simulink model "pendel_polar"  (Simulink 7.0)
settings: Solver=ode45  StartTime=0.0  StopTime=tstop  FixedStep=0.8  MaxStep=0.8  RelTol=1e-6
values from neighbouring files (symbols this model uses):
  g = 9.81    [main_pendel_kartesisch.m]    (also in main_pendel_polar.m)
  l = 1    [main_pendel_kartesisch.m]    (also in main_pendel_polar.m)
  omega0 = 0    [main_pendel_polar.m]
  phi0 = 45 *pi/180    (= 0.785398163397)    [main_pendel_polar.m]
libraries: simulink x3
settings Model: Creator=adminus  LastModifiedBy=adminus
settings DataIOCC: OutputOption=SpecifiedOutputTimes  OutputTimes=[0:0.01:5]
settings OptimizationCC: BlockReduction=off
settings DebuggingCC: SaveWithParameterizedLinksMsg=none  SignalResolutionControl=TryResolveAllWithWarning  SolverPrmCheckMsg=none  MultiTaskDSMMsg=warning  MultiTaskCondExecSysMsg=none  StrictBusMsg=None
settings HardwareCC: TargetUnknown=on
settings RTWCC: IncludeERTFirstTime=on

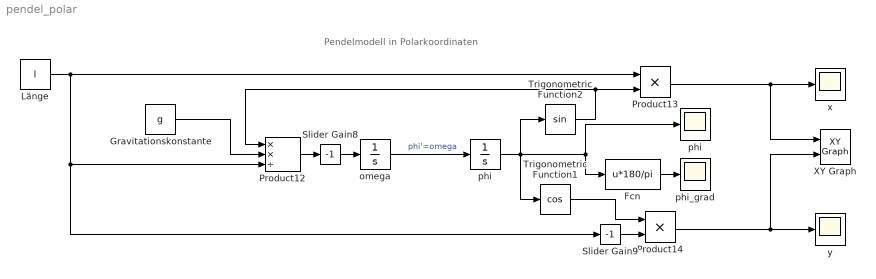
== system pendel_polar ==
  note: Pendelmodell in Polarkoordinaten
  Fcn : Fcn  Expr=u*180/pi
  Gravitationskonstante : Constant  Value=g
  Länge : Constant  Value=l
  Product12 : Product  Inputs=**/  SaturateOnIntegerOverflow=on  RndMeth=Zero  InputSameDT=on
  Product13 : Product  SaturateOnIntegerOverflow=on  RndMeth=Zero  InputSameDT=on
  Product14 : Product  SaturateOnIntegerOverflow=on  RndMeth=Zero  InputSameDT=on
  Slider Gain8 : simulink/Math Operations/Slider Gain  SystemSampleTime=-1  low=-1  gain=-1  high=2
  Slider Gain9 : simulink/Math Operations/Slider Gain  SystemSampleTime=-1  low=-1  gain=-1  high=2
  Trigonometric Function1 : Trigonometry  Operator=cos
  Trigonometric Function2 : Trigonometry
  XY Graph : simulink/Sinks/XY Graph  SystemSampleTime=-1  xmin=-1.1*l  xmax=1.1*l  ymin=-1.1*l  ymax=1.1*l  st=-1
  omega : Integrator  InitialCondition=omega0
  phi : Scope
  "phi " : Integrator  InitialCondition=phi0
  phi_grad : Scope
  x : Scope
      settings: SaveName=ScopeData2
  y : Scope
      settings: SaveName=ScopeData3
  wires:
  Gravitationskonstante/1 -> Product12/2
  Länge/1 -> Product13/1, Product12/3, Slider Gain9/1
  omega/1 -> "phi "/1  "phi'=omega"
  "phi "/1 -> Trigonometric Function2/1, Trigonometric Function1/1, phi/1, Fcn/1
  Product12/1 -> Slider Gain8/1
  Trigonometric Function1/1 -> Product14/1
  Trigonometric Function2/1 -> Product13/2, Product12/1
  Slider Gain8/1 -> omega/1
  Product13/1 -> x/1, XY Graph/1
  Product14/1 -> XY Graph/2, y/1
  Slider Gain9/1 -> Product14/2
  Fcn/1 -> phi_grad/1
